simulink model "controlePorVariasSintoniasPID"  (R2023a)
settings: Solver=VariableStepAuto  StartTime=0.0  StopTime=2800  RelTol=1e-3
values from neighbouring files (symbols this model uses):
  F2 = 6.32    [ConstantesCPQ23m.m]    (also in lugardasRaizes.m)
  K = J/(Tau*wn2)    [ConstantesCPQ23m.m]    (also in lugardasRaizes.m)
  qsi = (P/Tau)/(2*wn)    [ConstantesCPQ23m.m]    (also in lugardasRaizes.m)
  wn = sqrt(1/Tau)    [ConstantesCPQ23m.m]    (also in lugardasRaizes.m)
  wn2 = (1/Tau)    [ConstantesCPQ23m.m]    (also in lugardasRaizes.m)
settings Model: Creator=Estudo  LastModifiedBy=Estudo

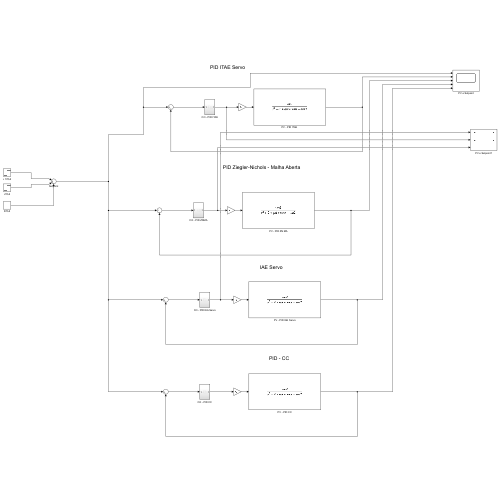
[thumbnail: Simulink's stored preview of the top-level diagram]
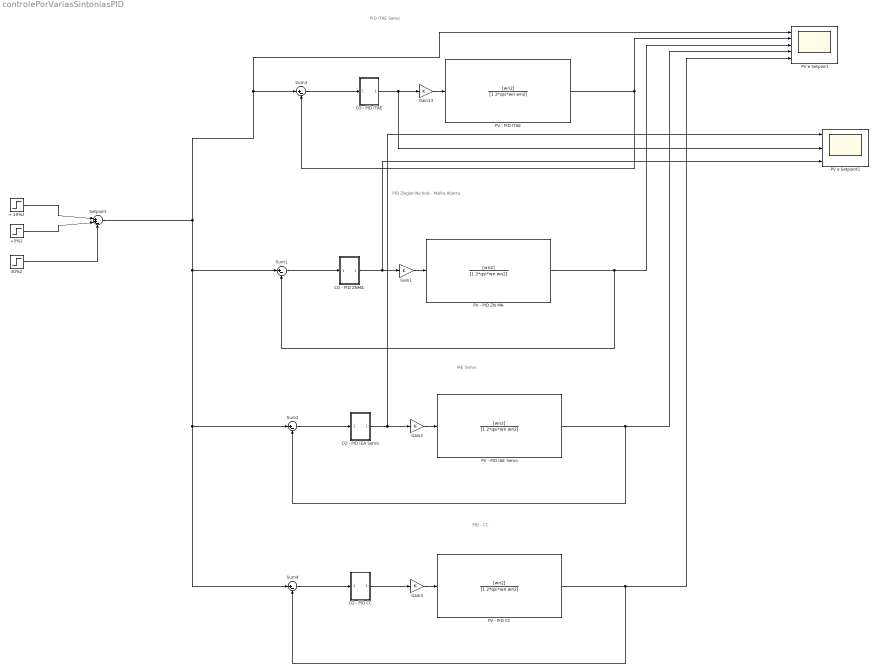
== system controlePorVariasSintoniasPID ==
  note: PID - CC
  note: IAE Servo
  note: PID Ziegler-Nichols - Malha Aberta
  note: PID ITAE Servo
  + 10%2 : Step  After=F2 + F2*0.1  SampleTime=0
  +5%2 : Step  Time=1200  After=F2*0.05  SampleTime=0
  30%2 : Step  Time=2000  After=F2*0.3  SampleTime=0
  CO - PID CC : Subsystem
  CO - PID IEA Servo : Subsystem
  CO - PID ITAE : Subsystem
  CO - PID ZNMA : Subsystem
  Gain{1..3,13} (4 alike) : Gain  Gain=K
  PV - PID CC : TransferFcn  Numerator=[wn2]  Denominator=[1 2*qsi*wn wn2]
  PV - PID IAE Servo : TransferFcn  Numerator=[wn2]  Denominator=[1 2*qsi*wn wn2]
  "PV - PID ITAE " : TransferFcn  Numerator=[wn2]  Denominator=[1 2*qsi*wn wn2]
  PV - PID ZN MA : TransferFcn  Numerator=[wn2]  Denominator=[1 2*qsi*wn wn2]
  PV e Setpoint : Scope  NumInputPorts=5
  PV e Setpoint1 : Scope  NumInputPorts=3
  Setpoint : Sum  Inputs=|++-
  Sum{1..4} (4 alike) : Sum  Inputs=|+-
  wires:
  30%2/1 -> Setpoint/3
  + 10%2/1 -> Setpoint/1
  +5%2/1 -> Setpoint/2
  PV - PID ZN MA/1 -> PV e Setpoint/3, Sum1/2
  Sum1/1 -> CO - PID ZNMA/1(In1)
  Gain1/1 -> PV - PID ZN MA/1
  Sum3/1 -> CO - PID ITAE/1(In1)
  Gain13/1 -> "PV - PID ITAE "/1
  CO - PID ITAE/1(Out1) -> PV e Setpoint1/2, Gain13/1
  PV - PID IAE Servo/1 -> PV e Setpoint/4, Sum2/2
  CO - PID IEA Servo/1(Out1) -> PV e Setpoint1/1, Gain2/1
  Sum2/1 -> CO - PID IEA Servo/1(In1)
  Gain2/1 -> PV - PID IAE Servo/1
  "PV - PID ITAE "/1 -> PV e Setpoint/2, Sum3/2
  CO - PID ZNMA/1(Out1) -> PV e Setpoint1/3, Gain1/1
  Sum4/1 -> CO - PID CC/1(In1)
  PV - PID CC/1 -> PV e Setpoint/5, Sum4/2
  Gain3/1 -> PV - PID CC/1
  Setpoint/1 -> PV e Setpoint/1, Sum3/1, Sum4/1, Sum2/1, Sum1/1
  CO - PID CC/1(Out1) -> Gain3/1

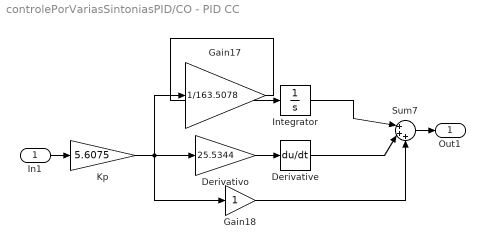
== system controlePorVariasSintoniasPID/CO - PID CC ==
  In1 : Inport
  Derivative : Derivative
  Derivativo : Gain  Gain=25.5344
  Gain17 : Gain  Gain=1/163.5078
  Gain18 : Gain
  Integrator : Integrator
  Kp : Gain  Gain=5.6075
  Sum7 : Sum  Inputs=|+++
  Out1 : Outport
  wires:
  Gain18/1 -> Sum7/3
  Integrator/1 -> Sum7/1
  Kp/1 -> Gain17/1, Gain18/1, Derivativo/1
  Derivativo/1 -> Derivative/1
  In1/1 -> Kp/1
  Gain17/1 -> Integrator/1
  Derivative/1 -> Sum7/2
  Sum7/1 -> Out1/1

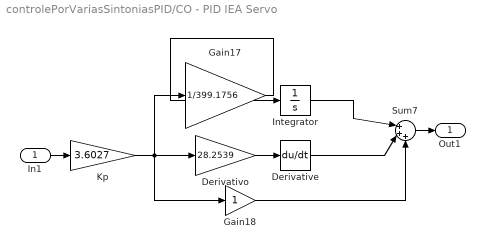
== system controlePorVariasSintoniasPID/CO - PID IEA Servo ==
  In1 : Inport
  Derivative : Derivative
  Derivativo : Gain  Gain=28.2539
  Gain17 : Gain  Gain=1/399.1756
  Gain18 : Gain
  Integrator : Integrator
  Kp : Gain  Gain=3.6027
  Sum7 : Sum  Inputs=|+++
  Out1 : Outport
  wires:
  Gain18/1 -> Sum7/3
  Integrator/1 -> Sum7/1
  Kp/1 -> Gain17/1, Gain18/1, Derivativo/1
  Derivativo/1 -> Derivative/1
  In1/1 -> Kp/1
  Gain17/1 -> Integrator/1
  Derivative/1 -> Sum7/2
  Sum7/1 -> Out1/1

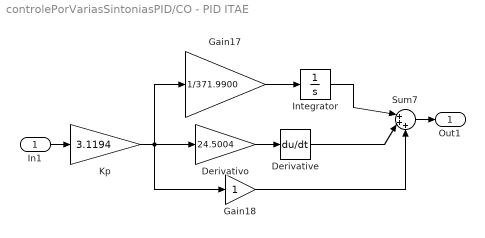
== system controlePorVariasSintoniasPID/CO - PID ITAE ==
  In1 : Inport
  Derivative : Derivative
  Derivativo : Gain  Gain=24.5004
  Gain17 : Gain  Gain=1/371.9900
  Gain18 : Gain
  Integrator : Integrator
  Kp : Gain  Gain=3.1194
  Sum7 : Sum  Inputs=|+++
  Out1 : Outport
  wires:
  Gain18/1 -> Sum7/3
  Integrator/1 -> Sum7/1
  Kp/1 -> Gain18/1, Gain17/1, Derivativo/1
  Derivativo/1 -> Derivative/1
  In1/1 -> Kp/1
  Gain17/1 -> Integrator/1
  Derivative/1 -> Sum7/2
  Sum7/1 -> Out1/1

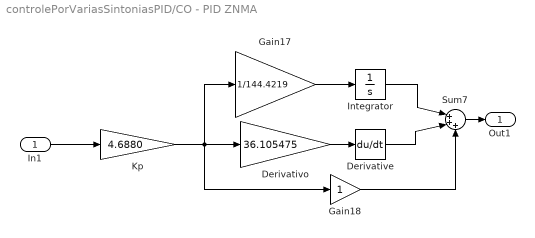
== system controlePorVariasSintoniasPID/CO - PID ZNMA ==
  In1 : Inport
  Derivative : Derivative
  Derivativo : Gain  Gain=36.105475
  Gain17 : Gain  Gain=1/144.4219
  Gain18 : Gain
  Integrator : Integrator
  Kp : Gain  Gain=4.6880
  Sum7 : Sum  Inputs=|+++
  Out1 : Outport
  wires:
  Gain18/1 -> Sum7/3
  Integrator/1 -> Sum7/1
  Kp/1 -> Gain17/1, Derivativo/1, Gain18/1
  Derivativo/1 -> Derivative/1
  In1/1 -> Kp/1
  Gain17/1 -> Integrator/1
  Derivative/1 -> Sum7/2
  Sum7/1 -> Out1/1
